simulink model "ex1_dummy"  (R2022a)
settings: Solver=VariableStepAuto  StartTime=0.0  StopTime=10.0  RelTol=1e-3
settings Model: Creator=Filippo  LastModifiedBy=Filippo

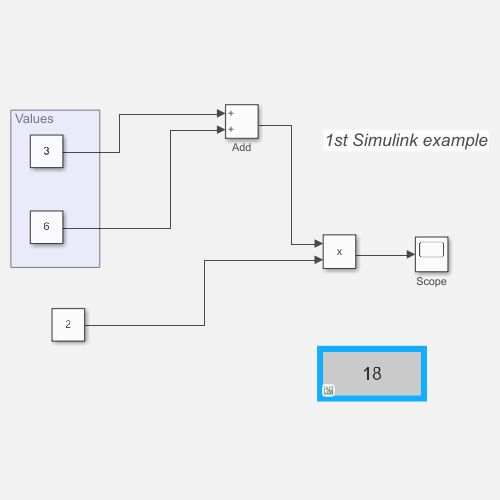
[thumbnail: Simulink's stored preview of the top-level diagram]
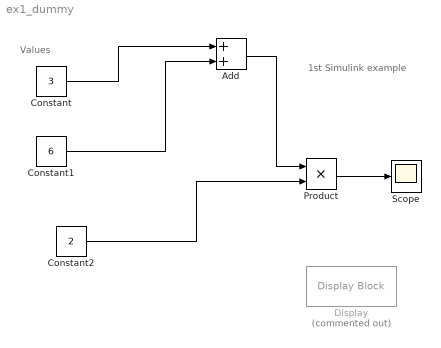
== system ex1_dummy ==
  note: Values
  note: 1st Simulink example
  Add : Sum
  Constant : Constant  Value=3
  Constant1 : Constant  Value=6
  Constant2 : Constant  Value=2
  Display : DisplayBlock  Commented=on  LabelPosition=Hide  Transparency=1
  Product : Product
  Scope : Scope
  wires:
  Constant/1 -> Add/1
  Constant1/1 -> Add/2
  Add/1 -> Product/1
  Constant2/1 -> Product/2
  Product/1 -> Scope/1
